simulink model "uav_model"  (R2025b)
settings: Solver=FixedStepAuto  StartTime=0.0  StopTime=100  FixedStep=0.01  RelTol=1e-3
InitFcn:
  | run('init_clicked_target_vars.m')
model workspace (MAT data in the model file):
  TGTCoordination = [50; 0; 0]
undefined symbols (not defined in the file or in its folder): Sim3dSensor, updateLatestCameraAimPoint, updateLatestSimFrameFromVector, updateLatestUavPos
libraries: sim3dlib x3, matrix_library x3, uavalgslib x2, uavsim3dlib x1, sim3dcameralib x1, visionsinks x1
settings Model: DataDictionary=fixedWingPathFollowingData.sldd  EnableAccessToBaseWorkspace=off  PacingRate=10  Creator=The MathWorks, Inc.  LastModifiedBy=2norm
settings SolverCC: AlgebraicLoopSolver=TrustRegion  DecoupledContinuousIntegration=on
settings DataIOCC: ReturnWorkspaceOutputs=off
settings DebuggingCC: UnconnectedInputMsg=warning  UnconnectedOutputMsg=warning  UnconnectedLineMsg=warning  ArithmeticOperatorsInVariantConditions=warning
settings ModelReferenceCC: EnableRefExpFcnMdlSchedulingChecks=on
settings SFSimCC: SimUseLocalCustomCode=off  CustomCodeUndefinedFunction=UseInterfaceOnly
settings RTWCC: RTWUseLocalCustomCode=off  GPUComputeCapability=3.5  DLArmComputeVersion=19.05

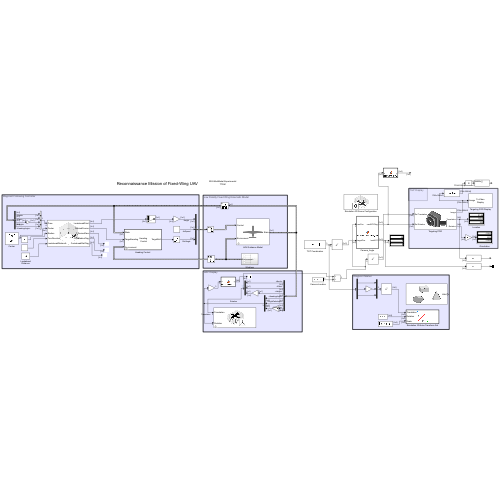
[thumbnail: Simulink's stored preview of the top-level diagram]
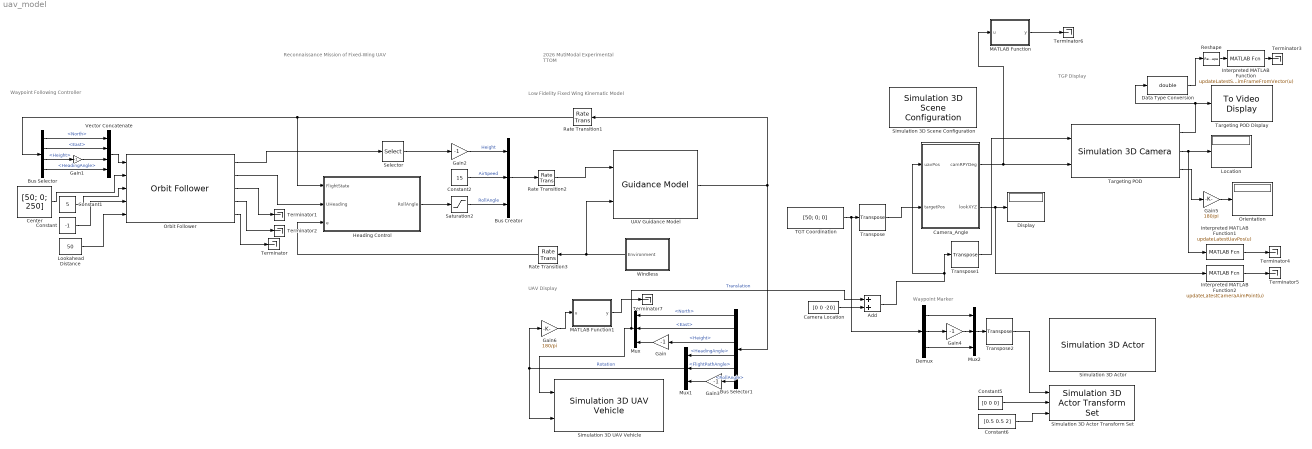
== system uav_model ==
  note: TGP Display
  note: Waypoint Marker
  note: UAV Display
  note: Reconnaissance Mission of Fixed-Wing UAV
  note: Low Fidelity Fixed Wing Kinematic Model
  note: Waypoint Following Controller
  note: 2026 MutiModal Experimental
      | TTOM
  Add : Sum
  Bus Creator : BusCreator  Inputs=3  OutDataTypeStr=Bus: FixedWingControlBus  NonVirtualBus=on
  Bus Selector : BusSelector  OutputSignals=North,East,Height,HeadingAngle
  Bus Selector1 : BusSelector  OutputSignals=North,East,Height,HeadingAngle,FlightPathAngle,RollAngle
  Camera Location : Constant  Value=[0 0 -20]
  Camera_Angle : MATLAB Function  TreatAsAtomicUnit=on
  Center : Constant  Value=[50; 0; 250]  VectorParams1D=off
  Constant : Constant  Value=-1
  Constant1 : Constant  Value=5
  Constant2 : Constant  Value=15
  Constant5 : Constant  Value=[0 0 0]  VectorParams1D=off
  Constant6 : Constant  Value=[0.5 0.5 2]  VectorParams1D=off
  Data Type Conversion : DataTypeConversion  OutDataTypeStr=double  SaturateOnIntegerOverflow=off  RndMeth=Floor
  Demux : Demux  Outputs=3
  Display : Display
  Gain{,1..4} (5 alike) : Gain  Gain=-1
  Gain5 : Gain  Gain=180/pi
  Gain6 : Gain  Gain=180/pi
  Heading Control : MATLAB Function  TreatAsAtomicUnit=on  mask(Fixed Wing Heading Controller){PHeadingAngle=3.530249625561657}
      mask prompts: PHeadingAngle "Heading Control Gain"
      mask help: P controller that regulates fixed wing UAV heading direction through controlling its roll angle. This controller requires that the plane is flying under coordinated flight condition.
  Interpreted MATLAB Function : MATLABFcn  MATLABFcn=updateLatestSimFrameFromVector(u)
  Interpreted MATLAB Function1 : MATLABFcn  MATLABFcn=updateLatestUavPos(u)
  Interpreted MATLAB Function2 : MATLABFcn  MATLABFcn=updateLatestCameraAimPoint(u)
  Location : Display
  Lookahead Distance : Constant  Value=50
  MATLAB Function : MATLAB Function  TreatAsAtomicUnit=on
  MATLAB Function1 : MATLAB Function  TreatAsAtomicUnit=on
  Mux : Mux  Inputs=3
  Mux1 : Mux  Inputs=3
  Mux2 : Mux  Inputs=3
  Orbit Follower : uavalgslib/Orbit Follower  UAVType=fixed-wing  MinOrbitRadius=5  MinLookaheadDistance=1  ExternalReset=none  ShowCrossTrackErrorOutput=off  ShowNumTurnsOutput=off  SimulateUsing=Interpreted execution
  Orientation : Display
  Rate Transition1 : RateTransition  OutPortSampleTime=0.01
  Rate Transition2 : RateTransition  OutPortSampleTime=0.1
  Rate Transition3 : RateTransition  OutPortSampleTime=0.01
  Reshape : Reshape  OutputDimensionality=Customize  OutputDimensions=[2764800 1]
  Saturation2 : Saturate  UpperLimit=20/180*pi  LowerLimit=-20/180*pi
  Selector : Selector  InputPortWidth=3  IndexOptions=Index vector (dialog)  Indices=[3]  OutputSizes=1
  Simulation 3D Actor : sim3dlib/Simulation 3D Actor  Priority=1  ActorName=Sim3dActor1  ParentName=Scene Origin  Operation=Create at setup  InitScriptText=|  SampleTime=-1  Translation=[0 0 0]  Rotation=[0 0 0]  Scale=[1 1 1]  aMode=5  ActorTag=Sim3dActor1  ActorType=Sim3dActor  ID=1
      | % Reserved keywords:
      | % Actor : handle to this actor object
      | % World : handle to the world object
      | 
      | % --- Create geometry once ---
      | if ~isprop(Actor, 'UserData') || isempty(Actor.UserData) || ~isfield(Actor.UserData,'markerCreated') || ~Actor.UserData.markerCreated
      |     % 원뿔 생성
      |     % 일반적으로 [radius height] 형식으로 쓰는 경우가 많음
      |     createShape(Actor, 'cone', [20 20 20]);
      | 
      |     % 색 지정
      |     Actor.Color = [1 0 0];   % red
      | 
      |     % 물리 비활성
      |     Actor.Physics = false;
      | 
      |     % 플래그 저장
      |     ud = struct();
      |     ud.markerCreated = true;
      |     Actor.UserData = ud;
      | end
  Simulation 3D Actor Transform Set : sim3dlib/Simulation 3D Actor Transform Set  Priority=-1  ActorTag=Sim3dActor1  CoordinateSystem=Default  NumberOfParts=1  CustNumOfParts=3  Translation=[50 0 -2]  Rotation=[0 0 0]  Scale=[0.5 0.5 2]  Ts=-1  aMode=0
      settings: LibrarySourceBlock=aerolibsim3d/Simulation 3D Actor Transform Set
  Simulation 3D Scene Configuration : sim3dlib/Simulation 3D Scene Configuration  Priority=0  ProjectFormat=Default Scenes  SceneDesc=Suburban scene  ProjectName=C:\Program Files\MATLAB\R2025b\toolbox\shared\sim3d_projects\automotive_project_windows\UE\WindowsNoEditor\VehicleSimulation.exe  ScenePath=/Game/Maps/HwStrght  EnableOpenDRIVE=off  vehTagList={'Custom';'Scene Origin';'Sim3dActor1';'SimulinkVehicle1'}  vehTag=SimulinkVehicle1  AttachedCameraRelativeTranslation=[0 0 300]  FreeCameraDefaultInitialTranslation=[-6, 0, 2]  AttachedCameraRelativeRotation=[0 0 0]  FreeCameraDefaultInitialRotation=[0, -15, 0]  ViewpointName=Custom  FreeCameraInitialTranslation=[-6 0 2]  ViewpointTranslation=[0 0 0]  FreeCameraInitialRotation=[0 -15 0]  ViewpointRotation=[0 0 0]  OpVisEn=off  Ts=.02  EnableWindow=on  EnableRemoteAccess=off  EnableWeather=off  SunAzimuth=90  SunAltitude=40.0  EnableGeospatialSun=off  Latitude=0  Longitude=0  Date=2023-01-01  Time=10:30:00  GeoTimeZone=-5.0  SunDaylightSaving=off  wind=1  clouds=10  EnableVolumetricClouds=off  CloudCoverage=0  CloudAltitude=6  fog=0  rain=0  RaindropsEffect=off  SnowDensity=0  EnableGeospatial=off  TilesetSource=Earth terrain  UseTrueOrigin=off  OriginHeight=200  OriginLatitude=40.744652  OriginLongitude=-73.988864  MapStyle=Aerial  AdditionalAssetIDs=[]  UseAdvancedSunSky=off  SolarTime=11  TimeZone=-5  Day=21  Month=9  Year=2022  UseDaylightSavingTime=on  DSTStartDay=10  DSTStartMonth=3  DSTEndDay=3  DSTEndMonth=11  DSTSwitchHour=2  sensorTag=MainCamera1  sensorId=1  sensorName=MainCamera1  mountLoc=Origin  offsetFlag=off  tmountOffset=[0, 0, 0]  rmountOffset=[0, 0, 0]  HorizontalResolution=1280  VerticalResolution=720  HorizontalFOV=60  mountPoint=[0 0 0]  mountOrientation=[0 0 0]  aMode=0  ID=1  GeoTrigger=Inactive  ViewNameList={'Custom'}  ViewTranslationList={'[-6 0 2]'}  ViewRotationList={'[0 -15 0]'}
      settings: LibrarySourceBlock=aerolibsim3d/Simulation 3D Scene Configuration
  Simulation 3D UAV Vehicle : uavsim3dlib/Simulation 3D UAV Vehicle  Priority=-1  Mesh=Fixed wing  MeshPath=/MathWorksUAVContent/UAVs/HexaRotorUAV/HexaRotor.HexaRotor  Color=Black  ActorName=SimulinkVehicle1  UseGlobalFrame=off  InitialTranslation=[0 0 0]  InitialRotation=[0 0 0]  InitialTranslationGlobal=[0 0 0]  InitialGeoOrigin=[0 0 0]  InitialRotationGlobal=[0 0 0]  SampleTime=-1  ActorType=SimulinkVehicle  ID=1  aMode=4  ActorTag=SimulinkVehicle1
  TGT Coordination : Constant  InitFcn=run('init_clicked_target_vars.m')  Value=[50; 0; 0]  OutDataTypeStr=double
  Targeting POD : sim3dcameralib/Simulation 3D Camera  Priority=1  sensorTag=Sim3dSensor�  sensorId=1  sensorName=Sim3dSensor�  vehTagList={'Scene Origin';'Sim3dActor1';'SimulinkVehicle1'}  vehTag=Scene Origin  CoordinateSystem=ISO8855  mountLoc=Origin  offsetFlag=on  tmountOffset=[0, 0, 0]  extTmount=on  rmountOffset=[0, 0, 0]  extRmount=on  FocalLength=[1109, 1109]  OpticalCenter=[640, 360]  ImageSize=[720, 1280]  RadialDistortion=[0, 0]  TangentialDistortion=[0, 0]  SensorSkew=0  VisualizeFieldOfView=off  FieldOfViewRange=300  DepthOutportEnabled=off  SemanticOutportEnabled=off  TransformOutportEnabled=on  SampleTime=-1  mountPoint=[0 0 0]  mountOrientation=[0 0 0]  aMode=3  ID=1
      settings: LibrarySourceBlock=drivingsim3d/Simulation 3D Camera
  Targeting POD Display : visionsinks/To Video Display  windowSizeMode=Normal  openAtMdlStart=on  fullScreen=off  videoWindowX=536805376  videoWindowY=536805376  saveWindowSize=off  videoWindowWidth=1280  videoWindowHeight=720  inputColorFormat=RGB  inputType=Obsolete  imagePorts=One multidimensional signal  OutputDevice=On-screen video monitor  dataOrg=Column-major  isWindowOpen=off
  Terminator{,1..7} (8 alike) : Terminator
  Transpose : matrix_library/Transpose
  Transpose1 : matrix_library/Transpose
  Transpose2 : matrix_library/Transpose
  UAV Guidance Model : uavalgslib/Guidance Model  ModelType=FixedWingGuidance  NumInstances=1  SpecifiedDataType=double  SimulateUsing=Code generation  InitialWorldPositionMultirotor=[0; 0; 0]  InitialWorldVelocityMultirotor=[0; 0; 0]  InitialEulerZYXMultirotor=[0; 0; 0]  InitialBodyAngularRateRPYMultirotor=[0; 0; 0]  InitialThrustMultirotor=0  InitialNorthFixedWing=-50  InitialEastFixedWing=0  InitialHeightFixedWing=-250  InitialAirSpeedFixedWing=15  InitialHeadingAngleFixedWing=0  InitialFlightPathAngleFixedWing=0  InitialRollAngleFixedWing=0  InitialRollAngleRateFixedWing=0  PDRollMultirotor=[3402.97,116.67]  PDPitchMultirotor=[3402.97, 116.67]  PYawRateMultirotor=1950  PThrustMultirotor=3900  MassMultirotor=0.1  PHeightFixedWing=3.9  PHeadingAngleFixedWing=3.9  PFlightPathAngleFixedWing=39  PDRollFixedWing=[5.9414, 3.9]  PAirSpeedFixedWing=1  FlightPathAngleLimitsFixedWing=[-pi/6, pi/6]  StateBusName='FixedWingStateBus'  ControlBusName='FixedWingControlBus'  EnvironmentBusName='FixedWingEnvironmentBus'  DataType=double
  Vector Concatenate : Concatenate  NumInputs=4
  Windless : Subsystem  VariantControl=NoWind
  wires:
  Constant2/1 -> Bus Creator/2  "AirSpeed"
  Gain2/1 -> Bus Creator/1  "Height"
  Bus Creator/1 -> Rate Transition2/1
  Bus Selector/1 -> Vector Concatenate/1  "<North>"
  Bus Selector/2 -> Vector Concatenate/2  "<East>"
  Saturation2/1 -> Bus Creator/3  "RollAngle"
  Rate Transition1/1 -> Heading Control/1(FlightState), Bus Selector/1
  Rate Transition2/1 -> UAV Guidance Model/1
  Orbit Follower/2 -> Heading Control/2(UHeading)
  Orbit Follower/1 -> Selector/1
  Center/1 -> Orbit Follower/2
  Vector Concatenate/1 -> Orbit Follower/1
  Orbit Follower/3 -> Terminator1/1
  Lookahead Distance/1 -> Orbit Follower/5
  Heading Control/1(RollAngle) -> Saturation2/1
  Bus Selector1/6 -> Gain3/1  "<RollAngle>"
  Bus Selector1/5 -> Mux1/2  "<FlightPathAngle>"
  Mux1/1 -> Simulation 3D UAV Vehicle/2, Gain6/1  "Rotation"
  UAV Guidance Model/1 -> Bus Selector1/1, Rate Transition1/1
  Mux/1 -> Simulation 3D UAV Vehicle/1, Add/1  "Translation"
  Windless/1(Environment) -> UAV Guidance Model/2, Rate Transition3/1
  Bus Selector/4 -> Vector Concatenate/4  "<HeadingAngle>"
  Bus Selector/3 -> Gain1/1  "<Height>"
  Gain1/1 -> Vector Concatenate/3
  Selector/1 -> Gain2/1
  Rate Transition3/1 -> Heading Control/3(e)
  Bus Selector1/1 -> Mux/1  "<North>"
  Bus Selector1/2 -> Mux/2  "<East>"
  Bus Selector1/4 -> Mux1/1  "<HeadingAngle>"
  Bus Selector1/3 -> Gain/1  "<Height>"
  Orbit Follower/4 -> Terminator2/1
  Targeting POD/2 -> Interpreted MATLAB Function1/1, Location/1
  Targeting POD/3 -> Gain5/1
  Orbit Follower/5 -> Terminator/1
  Constant/1 -> Orbit Follower/4
  Constant1/1 -> Orbit Follower/3
  Targeting POD/1 -> Data Type Conversion/1, Targeting POD Display/1
  Camera_Angle/1(camRPYDeg) -> MATLAB Function/1(u), Targeting POD/2
  Gain5/1 -> Orientation/1
  Transpose1/1 -> Targeting POD/1
  Camera Location/1 -> Add/2
  Add/1 -> Camera_Angle/1(uavPos), Transpose1/1
  Gain/1 -> Mux/3
  Gain3/1 -> Mux1/3
  Camera_Angle/2(lookXYZ) -> Interpreted MATLAB Function2/1, Display/1
  Constant6/1 -> Simulation 3D Actor Transform Set/3
  Constant5/1 -> Simulation 3D Actor Transform Set/2
  TGT Coordination/1 -> Demux/1, Transpose/1
  Mux2/1 -> Transpose2/1
  Demux/1 -> Mux2/1
  Demux/2 -> Gain4/1
  Demux/3 -> Mux2/3
  Gain4/1 -> Mux2/2
  Transpose/1 -> Camera_Angle/2(targetPos)
  Transpose2/1 -> Simulation 3D Actor Transform Set/1
  Interpreted MATLAB Function/1 -> Terminator3/1
  Reshape/1 -> Interpreted MATLAB Function/1
  Data Type Conversion/1 -> Reshape/1
  Interpreted MATLAB Function1/1 -> Terminator4/1
  Interpreted MATLAB Function2/1 -> Terminator5/1
  MATLAB Function/1(y) -> Terminator6/1
  MATLAB Function1/1(y) -> Terminator7/1
  Gain6/1 -> MATLAB Function1/1(u)

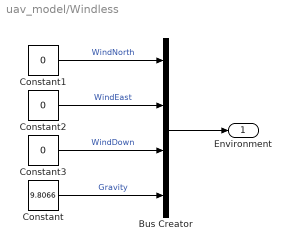
== system uav_model/Windless ==
  Bus Creator : BusCreator  Inputs=4  OutDataTypeStr=Bus: FixedWingEnvironmentBus  NonVirtualBus=on
  Constant : Constant  Value=9.8066
  Constant1 : Constant  Value=0
  Constant2 : Constant  Value=0
  Constant3 : Constant  Value=0
  Environment : Outport  VectorParamsAs1DForOutWhenUnconnected=off
  wires:
  Constant2/1 -> Bus Creator/2  "WindEast"
  Constant3/1 -> Bus Creator/3  "WindDown"
  Constant1/1 -> Bus Creator/1  "WindNorth"
  Bus Creator/1 -> Environment/1
  Constant/1 -> Bus Creator/4  "Gravity"

== matlab function uav_model/Camera_Angle ==
  data: uavPos input; targetPos input; camRPYDeg output; lookXYZ output
function [camRPYDeg, lookXYZ] = cameraWorldTrackNEU_NorthUp(uavPos, targetPos)
% cameraWorldTrackNEU_NorthUp
%
% Inputs
%   uavPos    : [N E U]
%   targetPos : [N E U]
%
% Outputs
%   camRPYDeg : [roll pitch yaw] in degree, world-referenced
%   lookXYZ   : [x y z] point where camera LOS intersects ground plane z=0
%
% Assumptions
%   - World frame is NEU: x=N, y=E, z=U
%   - Camera forward axis is +X
%   - Camera right axis   is +Y
%   - Camera up axis      is +Z
%   - Euler output uses ZYX order:
%       yaw about Z, pitch about Y, roll about X
%
% Goal
%   - Camera looks at target
%   - Screen top points toward North as much as possible

camRPYDeg = [0 0 0];
lookXYZ   = [0 0 0];

pu = uavPos(:);
pt = targetPos(:);

if numel(pu) ~= 3 || numel(pt) ~= 3
    return;
end

if ~all(isfinite(pu)) || ~all(isfinite(pt))
    return;
end

% Camera position
pc = pu;

% Forward axis: camera -> target
f = pt - pc;
nf = norm(f);
if nf < 1e-9
    return;
end
f = f / nf;

% Desired "screen up" reference = North
north_w = [1; 0; 0];

% Project north onto plane perpendicular to forward
u = north_w - dot(north_w, f) * f;
nu = norm(u);

% Singularity: if looking almost exactly north/south,
% projected north becomes too small.
% Fallback to world up.
if nu < 1e-9
    alt = [0; 0; 1];
    u = alt - dot(alt, f) * f;
    nu = norm(u);
    if nu < 1e-9
        return;
    end
end
u = u / nu;

% right = up x forward
r = cross(u, f);
nr = norm(r);
if nr < 1e-9
    return;
end
r = r / nr;

% re-orthogonalize up = forward x right
u = cross(f, r);
u = u / norm(u);

% Rotation from camera frame to world frame
R_cw = [f, r, u];

% Extract ZYX Euler angles
pitch = asin(-R_cw(3,1));
cp = cos(pitch);

if abs(cp) < 1e-9
    yaw  = atan2(-R_cw(1,2), R_cw(2,2));
    roll = 0;
else
    yaw  = atan2(R_cw(2,1), R_cw(1,1));
    roll = atan2(R_cw(3,2), R_cw(3,3));
end

camRPYDeg = [rad2deg(roll), rad2deg(pitch), rad2deg(yaw)];

% -------------------------------------------------
% Ground intersection of camera line-of-sight
% Ground plane: z = 0
% LOS: p(t) = pc + t*f, t >= 0
% Solve pc(3) + t*f(3) = 0
% -------------------------------------------------
groundPoint = pt;   % fallback

if abs(f(3)) > 1e-9
    t = -pc(3) / f(3);
    if t >= 0
        cand = pc + t * f;
        if all(isfinite(cand))
            groundPoint = cand;
        end
    end
end

lookXYZ = groundPoint.';

if ~all(isfinite(camRPYDeg))
    camRPYDeg = [0 0 0];
end

if ~all(isfinite(lookXYZ))
    lookXYZ = [0 0 0];
end

== matlab function uav_model/Heading Control ==
  data: FlightState input Bus: FixedWingStateBus; UHeading input; RollAngle output size=[1 1]; e input Bus: FixedWingEnvironmentBus; PHeadingAngle parameter
function RollAngle = fcn(FlightState, UHeading, e, PHeadingAngle)
    
    Va = FlightState.AirSpeed;
    HeadingAngle = FlightState.HeadingAngle;
    FlightPathAngle = FlightState.FlightPathAngle;
    
    YawAngle = HeadingAngle - asin((1/Va)*[e.WindNorth, e.WindEast]*[-sin(HeadingAngle); cos(HeadingAngle)]);
    b = [cos(HeadingAngle)*cos(FlightPathAngle), sin(HeadingAngle)*cos(FlightPathAngle), -sin(FlightPathAngle)]*[e.WindNorth; e.WindEast; e.WindDown];
    c = [e.WindNorth, e.WindEast, e.WindDown]*[e.WindNorth; e.WindEast; e.WindDown]- Va^2;
    Vg = -b+sqrt(b^2-c);
    
    RollAngle = atan2(PHeadingAngle*angdiff(HeadingAngle,UHeading)*Vg,e.Gravity*cos(HeadingAngle-YawAngle));

== matlab function uav_model/MATLAB Function ==
  data: u input; y output
function y = exportCamRPYDeg(u)
%#codegen
y = u;
coder.extrinsic('assignin');
assignin('base', 'latestCamRPYDeg', u);

== matlab function uav_model/MATLAB Function1 ==
  data: u input; y output
function y = exportGuidanceEulerDeg(u)
%#codegen
y = u;
coder.extrinsic('assignin');
assignin('base', 'latestGuidanceEulerDeg', u);
